simulink model "generate_cartesian_pose_motion"  (R2025a)
settings: Solver=FixedStepDiscrete  StartTime=0.0  StopTime=inf  FixedStep=0.001  RelTol=1e-3  EnableMultiTasking=on
PreLoadFcn:
  | frs = FrankaRobotSettings;
libraries: franka_simulink x1
settings Model: SimulationMode=external  ExtModeTrigDuration=10000  Creator=vasi_ko  LastModifiedBy=kvasios
settings SolverCC: AlgebraicLoopSolver=TrustRegion
settings DataIOCC: LimitDataPoints=on  SaveFormat=Array  ReturnWorkspaceOutputs=off
settings OptimizationCC: EnhancedBackFolding=on  PassReuseOutputArgsThreshold=0.0  OptimizeBlockOrder=speed  DifferentSizesBufferReuse=on  OptimizationCustomize=off
settings DebuggingCC: SolverPrmCheckMsg=warning  ParameterTunabilityLossMsg=error  UnconnectedInputMsg=warning  UnconnectedOutputMsg=warning  UnconnectedLineMsg=warning  SFUnexpectedBacktrackingDiag=warning  SFNoUnconditionalDefaultTransitionDiag=warning  SFExecutionAtInitializationDiag=none  ArithmeticOperatorsInVariantConditions=warning
settings HardwareCC: ProdBitPerLong=64.0  ProdHWDeviceType=Intel->x86-64 (Linux 64)
settings ModelReferenceCC: EnableRefExpFcnMdlSchedulingChecks=on  PropagateSignalLabelsOutOfModel=off
settings SFSimCC: SimUseLocalCustomCode=off  MATLABDynamicMemAlloc=off  CustomCodeUndefinedFunction=UseInterfaceOnly  SimTargetLang=C++  SimDLTargetLibrary=mkl-dnn
settings RTWCC: HardwareBoard=Generic Linux AMD64 Board  RTWVerbose=off  RTWUseLocalCustomCode=off  BuildConfiguration=Faster Runs  TargetLang=C++  GPUComputeCapability=3.5  DLArmComputeVersion=19.05
settings CodeAppCC: ForceParamTrailComments=on  OperatorAnnotations=on
settings GRTTargetCC: ExtMode=on  ExtModeStaticAlloc=on  ExtModeMexFile=ext_xcp  ExtModeIntrfLevel=Level2 - Open  TargetLangStandard=C++14 (ISO)
settings ConfigComp: CovMetricSettings=dw  CovSaveCumulativeToWorkspaceVar=on  CovSaveSingleToWorkspaceVar=on  CovExternalEMLEnable=off  CovSFcnEnable=off

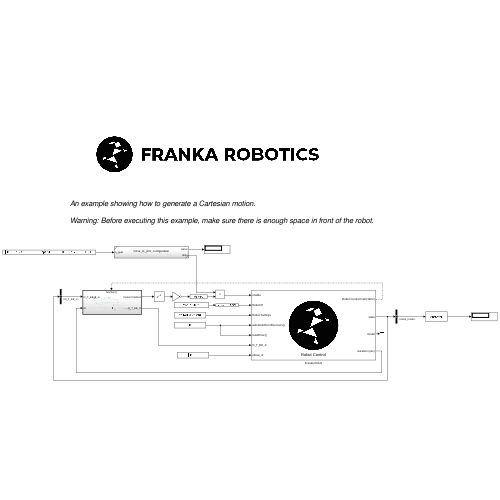
[thumbnail: Simulink's stored preview of the top-level diagram]
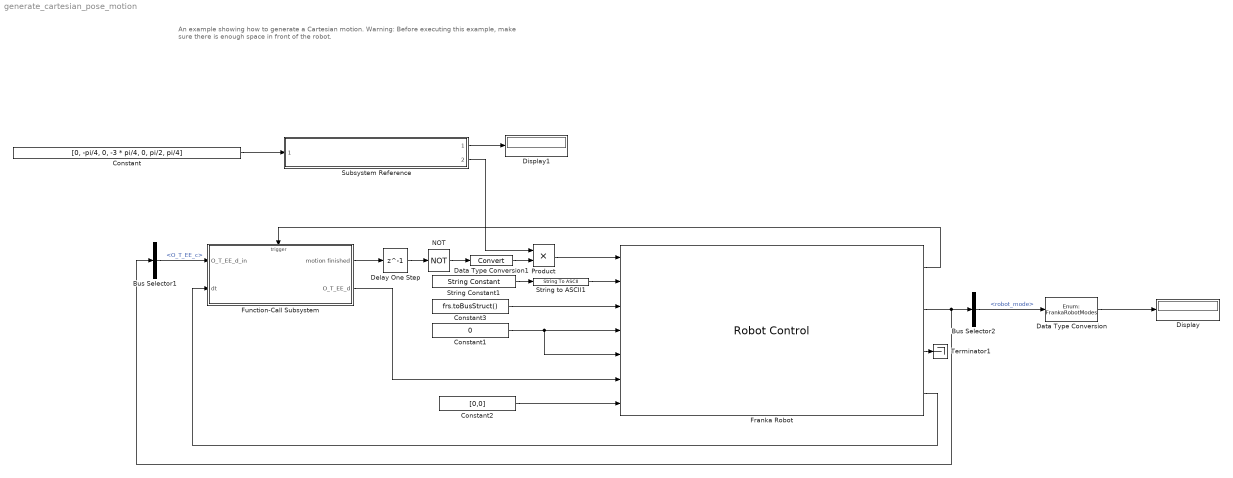
== system generate_cartesian_pose_motion ==
  note: An example showing how to generate a Cartesian motion.
      |
      | Warning: Before executing this example, make sure there is enough space in front of the robot.
  Bus Selector1 : BusSelector  OutputSignals=O_T_EE_c
  Bus Selector2 : BusSelector  OutputSignals=robot_mode
  Constant : Constant  Value=[0, -pi/4, 0, -3 * pi/4, 0, pi/2, pi/4]
  Constant1 : Constant  Value=0  OutDataTypeStr=Inherit: Inherit via back propagation
  Constant2 : Constant  Value=[0,0]  OutDataTypeStr=Inherit: Inherit via back propagation
  Constant3 : Constant  Value=frs.toBusStruct()  OutDataTypeStr=Bus: FrankaRobotSettingsBus
  Data Type Conversion : DataTypeConversion  OutDataTypeStr=Enum: FrankaRobotModes  SaturateOnIntegerOverflow=off  RndMeth=Floor
  Data Type Conversion1 : DataTypeConversion  SaturateOnIntegerOverflow=off  RndMeth=Floor
  Delay One Step : Delay  DelayLength=1
  Display : Display
  Display1 : Display
  Franka Robot : franka_simulink/Robot Control  control_mode=Cartesian Pose
      settings: SourceProductName=Franka Robotics Simulink Support Package
  Function-Call Subsystem : Subsystem  TreatAsAtomicUnit=on
      settings: RTWSystemCode=Nonreusable function
  NOT : Logic  Operator=NOT  IconShape=distinctive  AllPortsSameDT=off  OutDataTypeStr=boolean
  Product : Product
  String Constant1 : StringConstant  String="\"172.16.0.2\""
  String to ASCII1 : StringToASCII  OutputVectorSize=16
  Subsystem Reference : Subsystem  ReferencedSubsystem=move_to_joint_configuration
  Terminator1 : Terminator
  wires:
  Constant1/1 -> Franka Robot/5, Franka Robot/4
  String to ASCII1/1 -> Franka Robot/2
  Data Type Conversion/1 -> Display/1
  Subsystem Reference/1 -> Display1/1
  Function-Call Subsystem/2(O_T_EE_d) -> Franka Robot/6
  Bus Selector2/1 -> Data Type Conversion/1  "<robot_mode>"
  String Constant1/1 -> String to ASCII1/1
  Delay One Step/1 -> NOT/1
  Franka Robot/4 -> Function-Call Subsystem/2(dt)
  Franka Robot/1 -> Function-Call Subsystem/Trigger
  Constant3/1 -> Franka Robot/3
  NOT/1 -> Data Type Conversion1/1
  Subsystem Reference/2 -> Product/1
  Product/1 -> Franka Robot/1
  Constant/1 -> Subsystem Reference/1
  Franka Robot/2 -> Bus Selector1/1, Bus Selector2/1
  Data Type Conversion1/1 -> Product/2
  Bus Selector1/1 -> Function-Call Subsystem/1(O_T_EE_d_in)  "<O_T_EE_c>"
  Franka Robot/3 -> Terminator1/1
  Function-Call Subsystem/1(motion finished) -> Delay One Step/1
  Constant2/1 -> Franka Robot/7

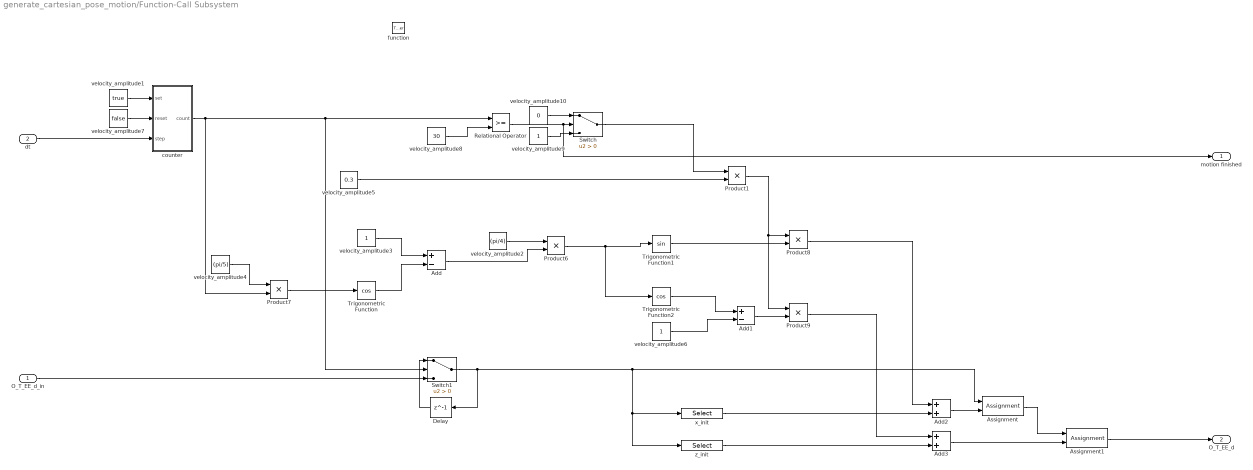
== system generate_cartesian_pose_motion/Function-Call Subsystem ==
  O_T_EE_d_in : Inport
  dt : Inport  Port=2
  function : TriggerPort  TriggerType=function-call  VariantControl=(inherit)
  Add : Sum  Inputs=+-
  Add1 : Sum  Inputs=+-
  Add2 : Sum
  Add3 : Sum
  Assignment : Assignment  NumberOfDimensions=2  DiagnosticForDimensions=Warning  IndexOptions=Index vector (dialog),Index vector (dialog)  Indices=1,4  OutputSizes=1,1
  Assignment1 : Assignment  NumberOfDimensions=2  DiagnosticForDimensions=Warning  IndexOptions=Index vector (dialog),Index vector (dialog)  Indices=3,4  OutputSizes=1,1
  Delay : Delay  DelayLength=1
  Product{1,6..9} (5 alike) : Product
  Relational Operator : RelationalOperator  OutDataTypeStr=boolean  InputSameDT=off
  Switch : Switch  Criteria=u2 > Threshold  SaturateOnIntegerOverflow=off  InputSameDT=off
  Switch1 : Switch  Criteria=u2 > Threshold  SaturateOnIntegerOverflow=off  InputSameDT=off
  Trigonometric Function : Trigonometry  Operator=cos  NumberOfIterations=50
  Trigonometric Function1 : Trigonometry  NumberOfIterations=50
  Trigonometric Function2 : Trigonometry  Operator=cos
  counter : Subsystem
  velocity_amplitude1 : Constant  Value=true  VectorParams1D=off
  velocity_amplitude10 : Constant  Value=0  VectorParams1D=off
  velocity_amplitude2 : Constant  Value=(pi/4)  VectorParams1D=off
  velocity_amplitude3 : Constant  VectorParams1D=off
  velocity_amplitude4 : Constant  Value=(pi/5)  VectorParams1D=off
  velocity_amplitude5 : Constant  Value=0.3  VectorParams1D=off
  velocity_amplitude6 : Constant  VectorParams1D=off
  velocity_amplitude7 : Constant  Value=false  VectorParams1D=off
  velocity_amplitude8 : Constant  Value=30  VectorParams1D=off
  velocity_amplitude9 : Constant  VectorParams1D=off
  x_init : Selector  NumberOfDimensions=2  InputPortWidth=16  IndexOptions=Index vector (dialog),Index vector (dialog)  Indices=1,4  OutputSizes=1,1
  z_init : Selector  NumberOfDimensions=2  InputPortWidth=16  IndexOptions=Index vector (dialog),Index vector (dialog)  Indices=3,4  OutputSizes=1,1
  motion finished : Outport  VectorParamsAs1DForOutWhenUnconnected=off
  O_T_EE_d : Outport  Port=2  VectorParamsAs1DForOutWhenUnconnected=off
  wires:
  Product8/1 -> Add2/1
  Relational Operator/1 -> motion finished/1, Switch/2
  Product6/1 -> Trigonometric Function1/1, Trigonometric Function2/1
  dt/1 -> counter/3(step)
  Switch/1 -> Product1/1
  z_init/1 -> Add3/2
  Assignment/1 -> Assignment1/1
  x_init/1 -> Add2/2
  Trigonometric Function/1 -> Add/2
  velocity_amplitude5/1 -> Product1/2
  velocity_amplitude1/1 -> counter/1(set)
  velocity_amplitude4/1 -> Product7/1
  velocity_amplitude9/1 -> Switch/3
  Add2/1 -> Assignment/2
  velocity_amplitude7/1 -> counter/2(reset)
  Product1/1 -> Product9/1, Product8/1
  Delay/1 -> Switch1/1
  Add1/1 -> Product9/2
  velocity_amplitude10/1 -> Switch/1
  Trigonometric Function1/1 -> Product8/2
  Switch1/1 -> Delay/1, z_init/1, x_init/1, Assignment/1
  velocity_amplitude3/1 -> Add/1
  O_T_EE_d_in/1 -> Switch1/3
  Product7/1 -> Trigonometric Function/1
  velocity_amplitude2/1 -> Product6/1
  Trigonometric Function2/1 -> Add1/1
  velocity_amplitude6/1 -> Add1/2
  Assignment1/1 -> O_T_EE_d/1
  Product9/1 -> Add3/1
  velocity_amplitude8/1 -> Relational Operator/2
  counter/1(count) -> Product7/2, Relational Operator/1, Switch1/2
  Add3/1 -> Assignment1/2
  Add/1 -> Product6/2

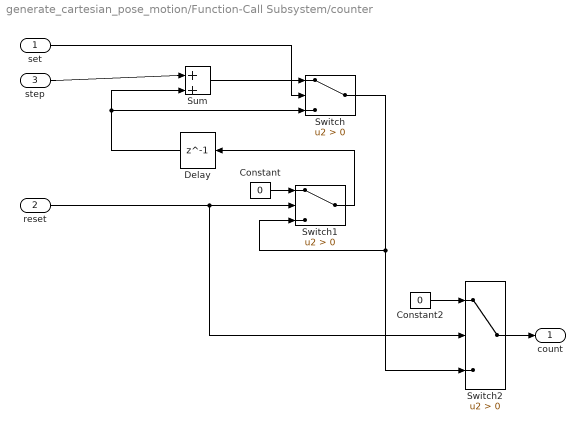
== system generate_cartesian_pose_motion/Function-Call Subsystem/counter ==
  set : Inport  OutDataTypeStr=boolean
  reset : Inport  Port=2  OutDataTypeStr=boolean
  step : Inport  Port=3  OutDataTypeStr=double
  Constant : Constant  Value=0  OutDataTypeStr=double
  Constant2 : Constant  Value=0  OutDataTypeStr=double
  Delay : Delay  DelayLength=1  InitialCondition=0
  Sum : Sum  Inputs=|++
  Switch : Switch  Criteria=u2 > Threshold  SaturateOnIntegerOverflow=off  InputSameDT=off
  Switch1 : Switch  Criteria=u2 > Threshold  OutDataTypeStr=double  SaturateOnIntegerOverflow=off  InputSameDT=off
  Switch2 : Switch  Criteria=u2 > Threshold  OutDataTypeStr=double  SaturateOnIntegerOverflow=off  InputSameDT=off
  count : Outport  OutDataTypeStr=double  VectorParamsAs1DForOutWhenUnconnected=off
  wires:
  Switch1/1 -> Delay/1
  Constant/1 -> Switch1/1
  reset/1 -> Switch2/2, Switch1/2
  Delay/1 -> Switch/3, Sum/2
  step/1 -> Sum/1
  Switch/1 -> Switch2/3, Switch1/3
  set/1 -> Switch/2
  Sum/1 -> Switch/1
  Constant2/1 -> Switch2/1
  Switch2/1 -> count/1
